simulink model "backup_of_step3"  (Simulink 10.2)
settings: Solver=ode113  StartTime=0.0  StopTime=5  RelTol=RT  AbsTol=AT  EnableMultiTasking=on
values from neighbouring files (symbols this model uses):
  Coefddq1 = polyfit(tv,ddq1d,5)    [TrajectoryPlanning_simulink.m]    (also in step2.mat = [4.72491967588e-15 -3.27046494167e-13 33.9277839628 -50.8916; step2_trajectory.m = polyfit(t_action,ddq1d,5); step3.m)
  Coefddq2 = polyfit(tv,ddq2d,5)    [TrajectoryPlanning_simulink.m]    (also in step2.mat = [9.35976668804e-13 -4.53899397056e-12 272.296235919 -408.444; step2_trajectory.m = polyfit(t_action,ddq2d,5); step3.m)
  Coefddq3 = polyfit(tv,ddq3d,5)    [TrajectoryPlanning_simulink.m]    (also in step2.mat = [-8.62483792285e-13 3.31083832504e-12 -180.560313738 270.840; step2_trajectory.m = polyfit(t_action,ddq3d,5); step3.m)
  Coefdq1 = polyfit(tv,dq1d,5)    [TrajectoryPlanning_simulink.m]    (also in step2.mat = [-5.68315943596e-14 8.48194599071 -16.9638919814 8.481945990; step2_trajectory.m = polyfit(t_action,dq1d,5); step3.m)
  Coefdq2 = polyfit(tv,dq2d,5)    [TrajectoryPlanning_simulink.m]    (also in step2.mat = [-5.14425222069e-13 68.0740589798 -136.14811796 68.074058979; step2_trajectory.m = polyfit(t_action,dq2d,5); step3.m)
  Coefdq3 = polyfit(tv,dq3d,5)    [TrajectoryPlanning_simulink.m]    (also in step2.mat = [8.05653713588e-13 -45.1400784346 90.2801568692 -45.14007843; step2_trajectory.m = polyfit(t_action,dq3d,5); step3.m)
  Coefq1 = polyfit(tv,q1d,5)    [TrajectoryPlanning_simulink.m]    (also in step2.mat = [1.69638919814 -4.24097299536 2.82731533024 7.50224544818e-1; step2_trajectory.m = polyfit(t_action,q1d,5); step3.m)
  Coefq2 = polyfit(tv,q2d,5)    [TrajectoryPlanning_simulink.m]    (also in step2.mat = [13.614811796 -34.0370294899 22.6913529933 -2.13681015439e-1; step2_trajectory.m = polyfit(t_action,q2d,5); step3.m)
  Coefq3 = polyfit(tv,q3d,5)    [TrajectoryPlanning_simulink.m]    (also in step2.mat = [-9.02801568692 22.5700392173 -15.0466928115 8.32884443522e-; step2_trajectory.m = polyfit(t_action,q3d,5); step3.m)
  F = [Fx;Fy;Mz]    [Jacobi_T.m]    (also in PRBDM_CTC_task.m = M_tilda*v+C_tilda*dX+G_tilda; RRR_CTC_task.m = M_tilda*v+V_tilda*dX+G_tilda; RRR_jtraj.m = q0; step2.mat = 10)
  gama0 = Rparams4dyn(3)    [PRBDM_3R_Dynamic_Matrices_Lagrange.m]    (also in PRBDM_3R_Dynamics.m = in4dyn(12); PRBDM_3R_Dynamics00.m = in4dyn(12); PRBDM_3R_DynamicsPID.m = in4dyn(12); PRBDM_3R_parameters.m = 0.1)
  gama1 = x(7)    [Jacobi_T.m]    (also in PRBDM_3R_Dynamic_Matrices_Lagrange.m = Rparams4dyn(4); PRBDM_3R_Dynamics.m = in4dyn(13); PRBDM_3R_Dynamics00.m = in4dyn(13); PRBDM_3R_DynamicsPID.m = in4dyn(13))
  gama2 = x(8)    [Jacobi_T.m]    (also in PRBDM_3R_Dynamic_Matrices_Lagrange.m = Rparams4dyn(5); PRBDM_3R_Dynamics.m = in4dyn(14); PRBDM_3R_Dynamics00.m = in4dyn(14); PRBDM_3R_DynamicsPID.m = in4dyn(14))
  gama3 = x(9)    [Jacobi_T.m]    (also in PRBDM_3R_Dynamic_Matrices_Lagrange.m = Rparams4dyn(6); PRBDM_3R_Dynamics.m = in4dyn(15); PRBDM_3R_Dynamics00.m = in4dyn(15); PRBDM_3R_DynamicsPID.m = in4dyn(15))
  k1 = Rparams4dyn(7)    [PRBDM_3R_Dynamic_Matrices_Lagrange.m]    (also in PRBDM_3R_Dynamics.m = in4dyn(16); PRBDM_3R_Dynamics00.m = in4dyn(16); PRBDM_3R_DynamicsPID.m = in4dyn(16); PRBDM_3R_parameters.m = 0.290628)
  k2 = Rparams4dyn(8)    [PRBDM_3R_Dynamic_Matrices_Lagrange.m]    (also in PRBDM_3R_Dynamics.m = in4dyn(17); PRBDM_3R_Dynamics00.m = in4dyn(17); PRBDM_3R_DynamicsPID.m = in4dyn(17); PRBDM_3R_parameters.m = 0.247572)
  k3 = Rparams4dyn(9)    [PRBDM_3R_Dynamic_Matrices_Lagrange.m]    (also in PRBDM_3R_Dynamics.m = in4dyn(18); PRBDM_3R_Dynamics00.m = in4dyn(18); PRBDM_3R_DynamicsPID.m = in4dyn(18); PRBDM_3R_parameters.m = 0.213624)
  kp = x(24)    [PRBDM_3R_CTC.m]    (also in PRBDM_3R_main.m = 20; PRBDM_3R_test001.m = 2; PRBDM_CTC_task.m = z(30); RRR_CTC.m)
  kv = x(23)    [PRBDM_3R_CTC.m]    (also in PRBDM_3R_main.m = 40; PRBDM_3R_test001.m = 4; PRBDM_CTC_task.m = z(29); RRR_CTC.m)
  L = Rparams4dyn(2)    [PRBDM_3R_Dynamic_Matrices_Lagrange.m]    (also in PRBDM_3R_Dynamics.m = in4dyn(11); PRBDM_3R_Dynamics00.m = in4dyn(11); PRBDM_3R_DynamicsPID.m = in4dyn(11); PRBDM_3R_parameters.m = 0.3)
  L0 = z(7)    [Forward_kinematics.m]    (also in GeometricCalculation_simulink.m = Geoparams(4); PRBDM_3R_parameters.m = 0.03; PRBDM_3R_parameters.mat = 0.03; TrajectoryPlanning_simulink.m = X(8))
  L1 = z(8)    [Forward_kinematics.m]    (also in GeometricCalculation_simulink.m = Geoparams(5); Jacobi.m = x(4); PRBDM_3R_CTC.m = x(19); PRBDM_3R_Dynamic_Matrices_NewtonEular.m = robot_params(4))
  L2 = z(9)    [Forward_kinematics.m]    (also in GeometricCalculation_simulink.m = Geoparams(6); Jacobi.m = x(5); PRBDM_3R_CTC.m = x(20); PRBDM_3R_Dynamic_Matrices_NewtonEular.m = robot_params(5))
  L3 = z(10)    [Forward_kinematics.m]    (also in GeometricCalculation_simulink.m = Geoparams(7); Jacobi.m = x(6); PRBDM_3R_CTC.m = x(21); PRBDM_3R_Dynamic_Matrices_NewtonEular.m = robot_params(6))
  m = Rparams4dyn(1)    [PRBDM_3R_Dynamic_Matrices_Lagrange.m]    (also in PRBDM_3R_Dynamics.m = in4dyn(10); PRBDM_3R_Dynamics00.m = in4dyn(10); PRBDM_3R_DynamicsPID.m = in4dyn(10); PRBDM_3R_parameters.m = 1)
  m1 = x(16)    [PRBDM_3R_CTC.m]    (also in PRBDM_3R_Dynamic_Matrices_NewtonEular.m = robot_params(1); PRBDM_3R_parameters.m = 0.35; PRBDM_3R_parameters.mat = 0.35; PRBDM_3R_test001.m = 0.1)
  m2 = x(17)    [PRBDM_3R_CTC.m]    (also in PRBDM_3R_Dynamic_Matrices_NewtonEular.m = robot_params(2); PRBDM_3R_parameters.m = 0.4; PRBDM_3R_parameters.mat = 0.4; PRBDM_3R_test001.m = 0.1)
  m3 = x(18)    [PRBDM_3R_CTC.m]    (also in PRBDM_3R_Dynamic_Matrices_NewtonEular.m = robot_params(3); PRBDM_3R_parameters.m = 0.15; PRBDM_3R_parameters.mat = 0.15; PRBDM_3R_test001.m = 0.1)
  Mz = x(6)    [Jacobi_T.m]    (also in step2.mat = 10; step2_trajectory.m = 10; step3.m = 10)
  phi = pi/3    (= 1.0471975512)    [PRBDM_3R_test001.m]
  t_action = [0 0.010101010101 0.020202020202 0.030303030303 0.040404040404 0.0505050505051 0.0606060606061 0.0707070707071 0.0808080808081 0.0909090909091 0.10101010101 0.111111111111 ... (100 elements, 1x100)]    [step2.mat]    (also in step2_trajectory.m = linspace(0,T_action,step); step3.m = 5)
  Theta_init = [0 0 0 0]    [step2.mat]    (also in step2_trajectory.m = [0     0     0     0    ]; step3.m = [0     0     0     0    ])
  W = x(22)    [PRBDM_3R_CTC.m]    (also in PRBDM_3R_Dynamic_Matrices_NewtonEular.m = robot_params(7); PRBDM_3R_Dynamics.m = in4dyn(20); PRBDM_3R_Dynamics00.m = in4dyn(20); PRBDM_3R_DynamicsPID.m = in4dyn(20))
  xd = 0.0536    [PRBDM_3R_test001.m]    (also in PRBDM_CTC_task.m = z(13); RRR_CTC_task.m = z(13))
  yd = 0.0135    [PRBDM_3R_test001.m]    (also in PRBDM_CTC_task.m = z(14); RRR_CTC_task.m = z(14))
settings Model: Creator=sayar  LastModifiedBy=Master
settings SolverCC: AutoScaleAbsTol=off
settings DataIOCC: SignalLoggingSaveFormat=Dataset  Refine=RF
settings OptimizationCC: ExpressionDepthLimit=2147483647
settings DebuggingCC: SolverPrmCheckMsg=warning  StateNameClashWarn=warning

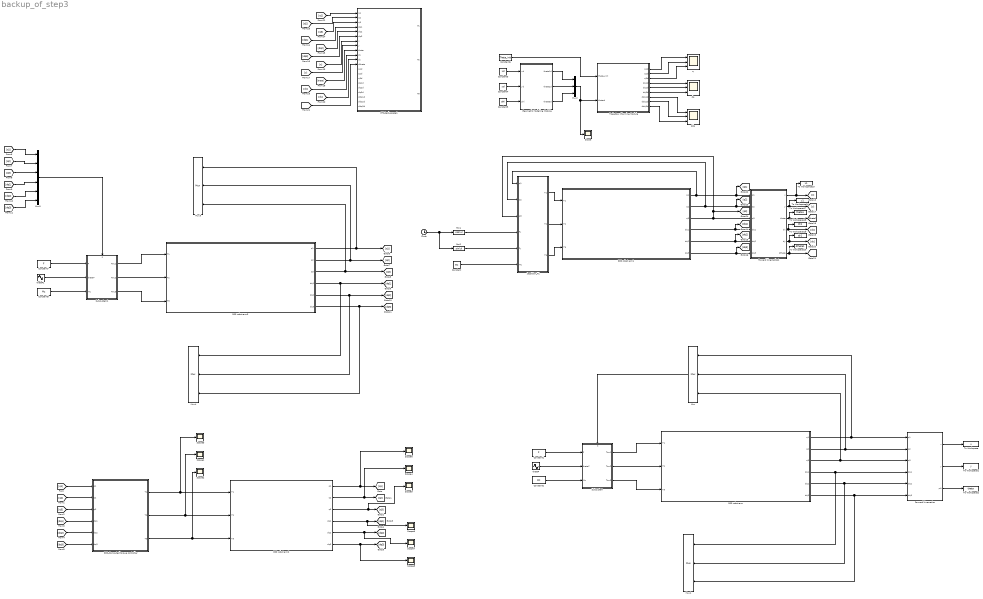
== system backup_of_step3 ==
  CTC_task_space1 : Subsystem
  Clock : Clock
  Constant : Constant  Value=Mz
  Constant1 : Constant  Value=F
  Constant2 : Constant  Value=Mz
  Constant3 : Constant  Value=xd
  Constant4 : Constant  Value=yd
  Constant5 : Constant  Value=phi
  Constant6 : Constant  Value=Theta_init
  Constant7 : Constant  Value=F
  Constant8 : Constant  Value=Mz
  Fcn1 : Fcn  Expr=cos(u)
  Fcn2 : Fcn  Expr=sin(u)
  Forward kinematics : Subsystem
  Forward kinematics1 : Subsystem
  Geometric Modeling Module : Subsystem
  Jacobian_T1 : Subsystem
  Mux{,1..4} (5 alike) : Mux  Inputs=3
  Mux5 : Mux  Inputs=6
  RRR robot arm : Subsystem
      mask Display: image(imread('RRR.png'))
  RRR robot arm1 : Subsystem
      mask Display: image(imread('RRR.png'))
  RRR robot arm2 : Subsystem
      mask Display: image(imread('RRR.png'))
  RRR robot arm3 : Subsystem
      mask Display: image(imread('RRR.png'))
  RRR_Computed torque controller : Subsystem
  Scope{,1..9} (10 alike) : Scope
  Subsystem : Subsystem
      settings: PortSchema="{\"entries\":[{\"content\":{\"sides\":[{\"content\":{\"connectorIds\":[\"In1\",\"In2\",\"In3\"]},\"type\":\"ConnectorPlacement.EquallySpacedRectSide\",\"uuid\":\"03e3fa68-98df-40a7-88fb-f274e89646de\"},{\"content\":{\"connectorIds\":[\"Out1\",\"Out2\",\"Out3\"],\"side\":\"RIGHT\"},\"type\":\"ConnectorPlacement.EquallySpacedRectSide\",\"uuid\":\"1a7c6e69-d785-4f03-b0d8-74a38f8f42a1\"},{\"content\":{\"connectorIds\":[\"In4\"],\"side\":\"TOP\"},\"type\":\"ConnectorPlacement.EquallySpacedRectSide\",\"uuid\":\"61c135cb-8cc5-493d-9c37-8230cda997e1\"},{\"content\":{\"connectorIds\":[],\"side\":\"HIDDEN\"},\"type\":\"ConnectorPlacement.EquallySpacedRectSide\",\"uuid\":\"5d99950e-feb6-474c-993a-cad470b06503\"}]},\"type\":\"ConnectorPlacement.EquallySpacedConnector\",\"uuid\":\"5533c5e9-db4a-4e3a-8115-8d67f8979e0c\"}],\"packageUris\":[\"http://schema.mathworks.com/mf0/Connector/R2020b\"],\"version\":\"1.0\"}"
  Subsystem1 : Subsystem
      settings: PortSchema="{\"entries\":[{\"content\":{\"sides\":[{\"content\":{\"connectorIds\":[\"In1\",\"In2\",\"In3\"]},\"type\":\"ConnectorPlacement.EquallySpacedRectSide\",\"uuid\":\"03e3fa68-98df-40a7-88fb-f274e89646de\"},{\"content\":{\"connectorIds\":[\"Out1\",\"Out2\",\"Out3\"],\"side\":\"RIGHT\"},\"type\":\"ConnectorPlacement.EquallySpacedRectSide\",\"uuid\":\"1a7c6e69-d785-4f03-b0d8-74a38f8f42a1\"},{\"content\":{\"connectorIds\":[\"In4\"],\"side\":\"TOP\"},\"type\":\"ConnectorPlacement.EquallySpacedRectSide\",\"uuid\":\"61c135cb-8cc5-493d-9c37-8230cda997e1\"},{\"content\":{\"connectorIds\":[],\"side\":\"HIDDEN\"},\"type\":\"ConnectorPlacement.EquallySpacedRectSide\",\"uuid\":\"5d99950e-feb6-474c-993a-cad470b06503\"}]},\"type\":\"ConnectorPlacement.EquallySpacedConnector\",\"uuid\":\"5533c5e9-db4a-4e3a-8115-8d67f8979e0c\"}],\"packageUris\":[\"http://schema.mathworks.com/mf0/Connector/R2020b\"],\"version\":\"1.0\"}"
  To Workspace : ToWorkspace  VariableName=x  SampleTime=-1
  To Workspace1 : ToWorkspace  VariableName=y  SampleTime=-1
  To Workspace15 : ToWorkspace  VariableName=x1  SampleTime=-1
  To Workspace16 : ToWorkspace  VariableName=y1  SampleTime=-1
  To Workspace17 : ToWorkspace  VariableName=theta1  SampleTime=-1
  To Workspace18 : ToWorkspace  VariableName=dx1  SampleTime=-1
  To Workspace19 : ToWorkspace  VariableName=dy1  SampleTime=-1
  To Workspace2 : ToWorkspace  VariableName=theta  SampleTime=-1
  To Workspace20 : ToWorkspace  VariableName=dtheta1  SampleTime=-1
  Trajectory Planning Module : Subsystem
  ddq : Scope  NumInputPorts=3
  dq : Scope  NumInputPorts=3
  q : Scope  NumInputPorts=3
  thetaF : Sin  SampleTime=0
  thetaF1 : Sin  SampleTime=0
  wires:
  Mux2/1 -> Scope/1, Trajectory Planning Module/2(thetad)
  Geometric Modeling Module/1(theta1d) -> Mux2/1
  Geometric Modeling Module/2(theta2d) -> Mux2/2
  Constant3/1 -> Geometric Modeling Module/1(xd)
  Constant5/1 -> Geometric Modeling Module/3(phi)
  Geometric Modeling Module/3(theta3d) -> Mux2/3
  Constant4/1 -> Geometric Modeling Module/2(yd)
  [y] -> CTC_task_space1/8(y)
  Forward kinematics1/6(dtheta) -> To Workspace20/1, [dtheta]
  Forward kinematics1/1(x) -> To Workspace15/1, [x]
  [dx] -> CTC_task_space1/10(dx)
  Forward kinematics1/3(theta) -> To Workspace17/1, [theta]
  RRR robot arm1/1(q1) -> [q1], Forward kinematics1/1(q1), Jacobian_T1/1(q1)
  [dy] -> CTC_task_space1/11(dy)
  RRR robot arm1/5(dq2) -> [dq2], Forward kinematics1/5(dq2)
  Jacobian_T1/3(T3) -> RRR robot arm1/3(T3)
  [dq2] -> CTC_task_space1/5(dq2)
  RRR robot arm1/6(dq3) -> [dq3], Forward kinematics1/6(dq3)
  [q1] -> CTC_task_space1/1(q1)
  [q3] -> CTC_task_space1/3(q3)
  [x] -> CTC_task_space1/7(x)
  [dq1] -> CTC_task_space1/4(dq1)
  Forward kinematics1/4(dx) -> To Workspace18/1, [dx]
  Forward kinematics1/2(y) -> To Workspace16/1, [y]
  Forward kinematics1/5(dy) -> To Workspace19/1, [dy]
  Jacobian_T1/2(T2) -> RRR robot arm1/2(T2)
  [dq3] -> CTC_task_space1/6(dq3)
  RRR robot arm1/4(dq1) -> [dq1], Forward kinematics1/4(dq1)
  [q2] -> CTC_task_space1/2(q2)
  Jacobian_T1/1(T1) -> RRR robot arm1/1(T1)
  RRR robot arm1/3(q3) -> Forward kinematics1/3(q3), [q3], Jacobian_T1/3(q3)
  [theta] -> CTC_task_space1/9(theta)
  [dtheta] -> CTC_task_space1/12(dtheta)
  RRR robot arm1/2(q2) -> [q2], Forward kinematics1/2(q2), Jacobian_T1/2(q2)
  Constant6/1 -> Trajectory Planning Module/1(theta_init)
  Trajectory Planning Module/1(q1d) -> q/1
  Trajectory Planning Module/2(q2d) -> q/2
  Trajectory Planning Module/3(q3d) -> q/3
  Trajectory Planning Module/4(dq1d) -> dq/1
  Trajectory Planning Module/5(dq2d) -> dq/2
  Trajectory Planning Module/6(dq3d) -> dq/3
  Trajectory Planning Module/8(ddq2d) -> ddq/2
  Trajectory Planning Module/9(ddq3d) -> ddq/3
  Trajectory Planning Module/7(ddq1d) -> ddq/1
  Clock/1 -> Fcn1/1, Fcn2/1
  Fcn2/1 -> Jacobian_T1/5(Fy)
  Fcn1/1 -> Jacobian_T1/4(Fx)
  Constant/1 -> Jacobian_T1/6(Mz)
  Mux/1 -> Subsystem/4(q)
  Subsystem/2(Tau2) -> RRR robot arm/2(T2)
  Subsystem/3(Tau3) -> RRR robot arm/3(T3)
  thetaF/1 -> Subsystem/2(thetaF)
  Forward kinematics/1(x) -> To Workspace/1
  Forward kinematics/3(phi) -> To Workspace2/1
  Forward kinematics/2(y) -> To Workspace1/1
  RRR robot arm/1(q1) -> Forward kinematics/1(q1), Mux/1
  Subsystem/1(Tau1) -> RRR robot arm/1(T1)
  RRR robot arm/2(q2) -> Mux/2, Forward kinematics/2(q2)
  RRR robot arm/6(dq3) -> Mux1/3, Forward kinematics/6(dq3)
  Constant2/1 -> Subsystem/3(Mz)
  RRR robot arm/5(dq2) -> Mux1/2, Forward kinematics/5(dq2)
  RRR robot arm/4(dq1) -> Mux1/1, Forward kinematics/4(dq1)
  RRR robot arm/3(q3) -> Mux/3, Forward kinematics/3(q3)
  Constant1/1 -> Subsystem/1(F)
  [dq3] -> RRR_Computed torque controller/6(dq3)
  RRR_Computed torque controller/1(T1) -> Scope3/1, RRR robot arm2/1(T1)
  [q3] -> RRR_Computed torque controller/3(q3)
  RRR robot arm2/5(dq2) -> Scope7/1, [dq2]
  RRR_Computed torque controller/2(T2) -> Scope1/1, RRR robot arm2/2(T2)
  RRR robot arm2/2(q2) -> Scope4/1, [q2]
  RRR robot arm2/4(dq1) -> Scope9/1, [dq1]
  RRR robot arm2/1(q1) -> Scope6/1, [q1]
  [dq1] -> RRR_Computed torque controller/4(dq1)
  [q2] -> RRR_Computed torque controller/2(q2)
  RRR robot arm2/6(dq3) -> Scope8/1, [dq3]
  [q1] -> RRR_Computed torque controller/1(q1)
  RRR_Computed torque controller/3(T3) -> Scope2/1, RRR robot arm2/3(T3)
  [dq2] -> RRR_Computed torque controller/5(dq2)
  RRR robot arm2/3(q3) -> Scope5/1, [q3]
  [dq3] -> Mux5/6
  [dq2] -> Mux5/5
  [q2] -> Mux5/2
  Subsystem1/3(Tau3) -> RRR robot arm3/3(T3)
  Subsystem1/2(Tau2) -> RRR robot arm3/2(T2)
  thetaF1/1 -> Subsystem1/2(thetaF)
  RRR robot arm3/6(dq3) -> [dq3], Mux4/3
  RRR robot arm3/2(q2) -> [q2], Mux3/2
  RRR robot arm3/1(q1) -> [q1], Mux3/1
  Subsystem1/1(Tau1) -> RRR robot arm3/1(T1)
  Constant7/1 -> Subsystem1/1(F)
  Constant8/1 -> Subsystem1/3(Mz)
  [q3] -> Mux5/3
  RRR robot arm3/5(dq2) -> [dq2], Mux4/2
  RRR robot arm3/4(dq1) -> [dq1], Mux4/1
  [q1] -> Mux5/1
  Mux5/1 -> Subsystem1/4(q)
  RRR robot arm3/3(q3) -> [q3], Mux3/3
  [dq1] -> Mux5/4

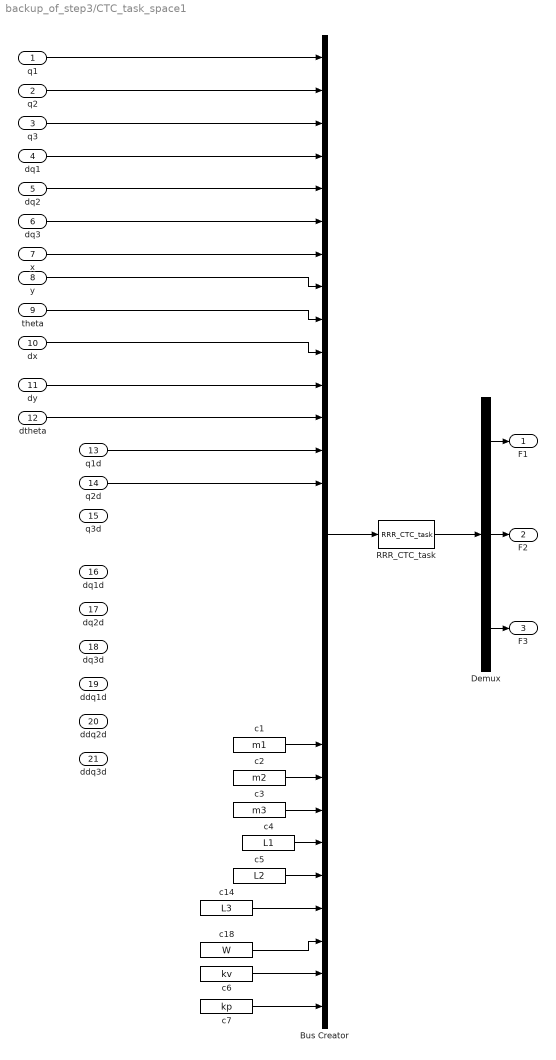
== system backup_of_step3/CTC_task_space1 ==
  q1 : Inport
  q2 : Inport  Port=2
  q3 : Inport  Port=3
  dq1 : Inport  Port=4
  dq2 : Inport  Port=5
  dq3 : Inport  Port=6
  x : Inport  Port=7
  y : Inport  Port=8
  theta : Inport  Port=9
  dx : Inport  Port=10
  dy : Inport  Port=11
  dtheta : Inport  Port=12
  q1d : Inport  Port=13
  q2d : Inport  Port=14
  q3d : Inport  Port=15
  dq1d : Inport  Port=16
  dq2d : Inport  Port=17
  dq3d : Inport  Port=18
  ddq1d : Inport  Port=19
  ddq2d : Inport  Port=20
  ddq3d : Inport  Port=21
  Bus Creator : BusCreator  Inputs=30
  Demux : Demux  Outputs=3
  RRR_CTC_task : MATLABFcn  MATLABFcn=RRR_CTC_task  OutputDimensions=3
  c1 : Constant  Value=m1
  c14 : Constant  Value=L3
  c18 : Constant  Value=W
  c2 : Constant  Value=m2
  c3 : Constant  Value=m3
  c4 : Constant  Value=L1
  c5 : Constant  Value=L2
  c6 : Constant  Value=kv
  c7 : Constant  Value=kp
  F1 : Outport
  F2 : Outport  Port=2
  F3 : Outport  Port=3
  wires:
  q3/1 -> Bus Creator/3
  RRR_CTC_task/1 -> Demux/1
  q1/1 -> Bus Creator/1
  Demux/3 -> F3/1
  q2/1 -> Bus Creator/2
  dq2/1 -> Bus Creator/5
  dq1/1 -> Bus Creator/4
  Demux/2 -> F2/1
  dq3/1 -> Bus Creator/6
  Demux/1 -> F1/1
  Bus Creator/1 -> RRR_CTC_task/1
  x/1 -> Bus Creator/7
  y/1 -> Bus Creator/8
  theta/1 -> Bus Creator/9
  dx/1 -> Bus Creator/10
  dy/1 -> Bus Creator/11
  dtheta/1 -> Bus Creator/12
  c1/1 -> Bus Creator/22
  c2/1 -> Bus Creator/23
  c3/1 -> Bus Creator/24
  c4/1 -> Bus Creator/25
  c5/1 -> Bus Creator/26
  c14/1 -> Bus Creator/27
  c18/1 -> Bus Creator/28
  c6/1 -> Bus Creator/29
  c7/1 -> Bus Creator/30
  q1d/1 -> Bus Creator/13
  q2d/1 -> Bus Creator/14

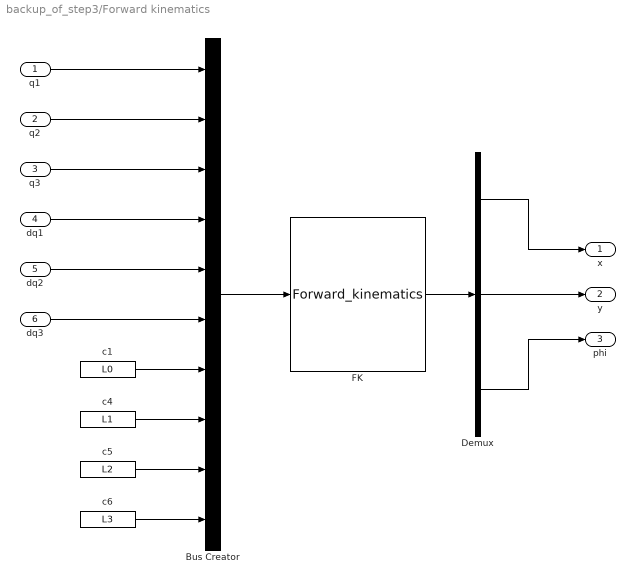
== system backup_of_step3/Forward kinematics ==
  q1 : Inport
  q2 : Inport  Port=2
  q3 : Inport  Port=3
  dq1 : Inport  Port=4
  dq2 : Inport  Port=5
  dq3 : Inport  Port=6
  Bus Creator : BusCreator  Inputs=10
  Demux : Demux  Outputs=3
  FK : MATLABFcn  MATLABFcn=Forward_kinematics  OutputDimensions=3
  c1 : Constant  Value=L0
  c4 : Constant  Value=L1
  c5 : Constant  Value=L2
  c6 : Constant  Value=L3
  x : Outport
  y : Outport  Port=2
  phi : Outport  Port=3
  wires:
  c6/1 -> Bus Creator/10
  Demux/1 -> x/1
  c4/1 -> Bus Creator/8
  q2/1 -> Bus Creator/2
  q1/1 -> Bus Creator/1
  q3/1 -> Bus Creator/3
  Bus Creator/1 -> FK/1
  dq2/1 -> Bus Creator/5
  Demux/2 -> y/1
  FK/1 -> Demux/1
  dq1/1 -> Bus Creator/4
  Demux/3 -> phi/1
  dq3/1 -> Bus Creator/6
  c5/1 -> Bus Creator/9
  c1/1 -> Bus Creator/7

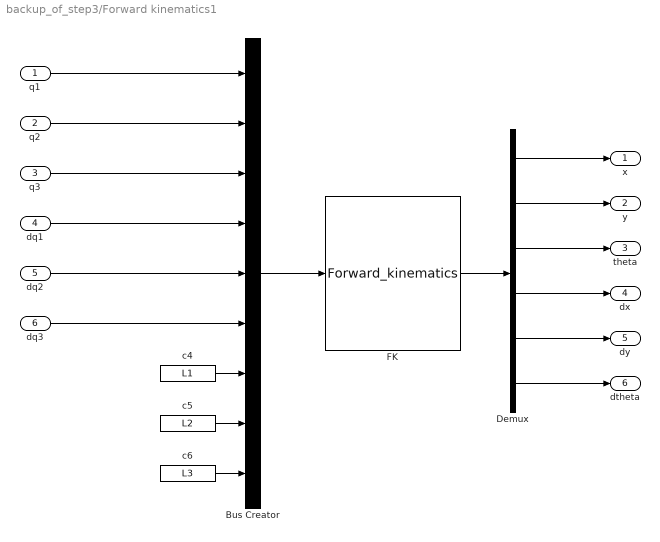
== system backup_of_step3/Forward kinematics1 ==
  q1 : Inport
  q2 : Inport  Port=2
  q3 : Inport  Port=3
  dq1 : Inport  Port=4
  dq2 : Inport  Port=5
  dq3 : Inport  Port=6
  Bus Creator : BusCreator  Inputs=9
  Demux : Demux  Outputs=6
  FK : MATLABFcn  MATLABFcn=Forward_kinematics  OutputDimensions=6
  c4 : Constant  Value=L1
  c5 : Constant  Value=L2
  c6 : Constant  Value=L3
  x : Outport
  y : Outport  Port=2
  theta : Outport  Port=3
  dx : Outport  Port=4
  dy : Outport  Port=5
  dtheta : Outport  Port=6
  wires:
  c6/1 -> Bus Creator/9
  Demux/1 -> x/1
  Demux/4 -> dx/1
  c4/1 -> Bus Creator/7
  Demux/5 -> dy/1
  q2/1 -> Bus Creator/2
  q1/1 -> Bus Creator/1
  q3/1 -> Bus Creator/3
  Bus Creator/1 -> FK/1
  dq2/1 -> Bus Creator/5
  Demux/2 -> y/1
  FK/1 -> Demux/1
  dq1/1 -> Bus Creator/4
  Demux/3 -> theta/1
  dq3/1 -> Bus Creator/6
  Demux/6 -> dtheta/1
  c5/1 -> Bus Creator/8

== system backup_of_step3/Geometric Modeling Module ==
  xd : Inport
  yd : Inport  Port=2
  phi : Inport  Port=3
  Demux : Demux  Outputs=3
  GeometricCalculation : MATLABFcn  MATLABFcn=GeometricCalculation_simulink
  Mux1 : Mux  Inputs=6
  c1 : Constant  Value=L0
  c2 : Constant  Value=L1
  c3 : Constant  Value=L2
  theta1d : Outport
  theta2d : Outport  Port=2
  theta3d : Outport  Port=3
  wires:
  Mux1/1 -> GeometricCalculation/1
  yd/1 -> Mux1/2
  xd/1 -> Mux1/1
  phi/1 -> Mux1/3
  c1/1 -> Mux1/4
  c3/1 -> Mux1/6
  c2/1 -> Mux1/5
  GeometricCalculation/1 -> Demux/1
  Demux/2 -> theta2d/1
  Demux/1 -> theta1d/1
  Demux/3 -> theta3d/1

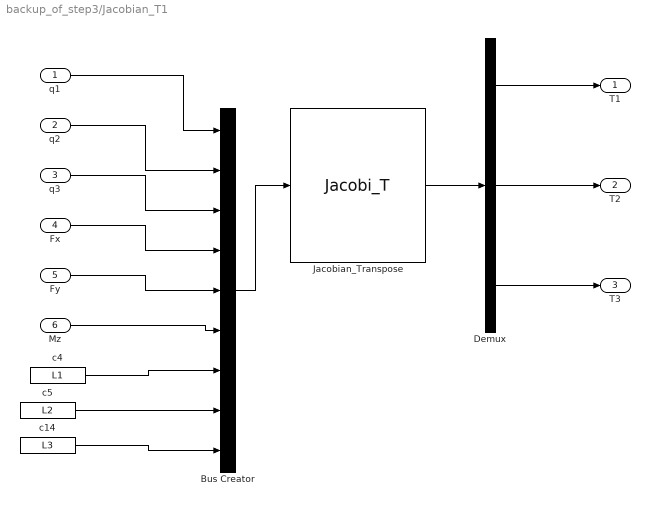
== system backup_of_step3/Jacobian_T1 ==
  q1 : Inport
  q2 : Inport  Port=2
  q3 : Inport  Port=3
  Fx : Inport  Port=4
  Fy : Inport  Port=5
  Mz : Inport  Port=6
  Bus Creator : BusCreator  Inputs=9
  Demux : Demux  Outputs=3
  Jacobian_Transpose : MATLABFcn  MATLABFcn=Jacobi_T  OutputDimensions=3
  c14 : Constant  Value=L3
  c4 : Constant  Value=L1
  c5 : Constant  Value=L2
  T1 : Outport
  T2 : Outport  Port=2
  T3 : Outport  Port=3
  wires:
  Jacobian_Transpose/1 -> Demux/1
  Demux/2 -> T2/1
  Bus Creator/1 -> Jacobian_Transpose/1
  Demux/1 -> T1/1
  Demux/3 -> T3/1
  Fx/1 -> Bus Creator/4
  Fy/1 -> Bus Creator/5
  Mz/1 -> Bus Creator/6
  q1/1 -> Bus Creator/1
  q2/1 -> Bus Creator/2
  q3/1 -> Bus Creator/3
  c5/1 -> Bus Creator/8
  c14/1 -> Bus Creator/9
  c4/1 -> Bus Creator/7

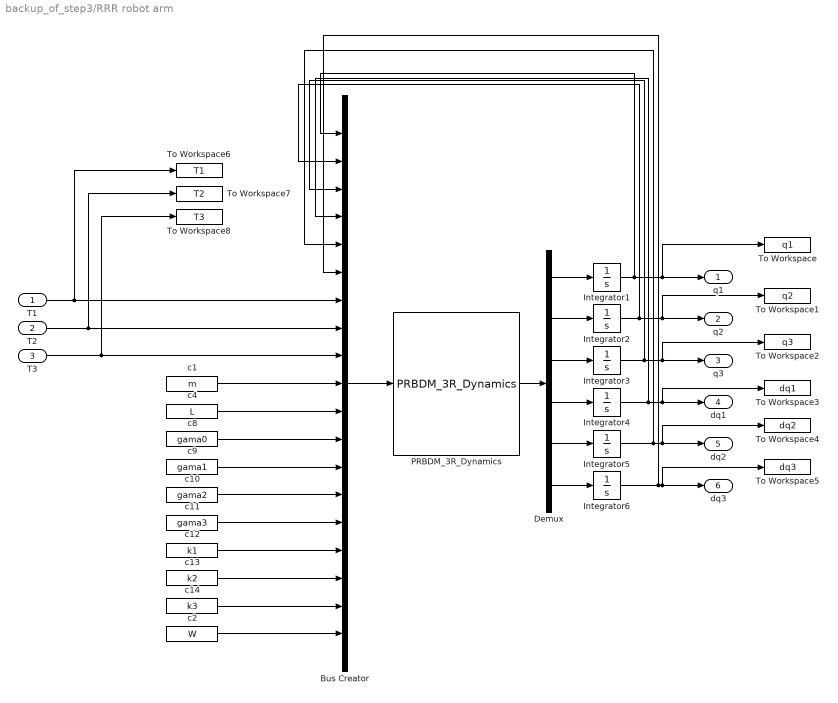
== system backup_of_step3/RRR robot arm ==
  T1 : Inport
  T2 : Inport  Port=2
  T3 : Inport  Port=3
  Bus Creator : BusCreator  Inputs=19
  Demux : Demux  Outputs=6
  Integrator{1,4..6} (4 alike) : Integrator
  Integrator2 : Integrator  InitialCondition=3*pi/4
  Integrator3 : Integrator  InitialCondition=-3*pi/4
  PRBDM_3R_Dynamics : MATLABFcn  MATLABFcn=PRBDM_3R_Dynamics  OutputDimensions=6
  To Workspace : ToWorkspace  VariableName=q1  SampleTime=-1
  To Workspace1 : ToWorkspace  VariableName=q2  SampleTime=-1
  To Workspace2 : ToWorkspace  VariableName=q3  SampleTime=-1
  To Workspace3 : ToWorkspace  VariableName=dq1  SampleTime=-1
  To Workspace4 : ToWorkspace  VariableName=dq2  SampleTime=-1
  To Workspace5 : ToWorkspace  VariableName=dq3  SampleTime=-1
  To Workspace6 : ToWorkspace  VariableName=T1  SampleTime=-1
  To Workspace7 : ToWorkspace  VariableName=T2  SampleTime=-1
  To Workspace8 : ToWorkspace  VariableName=T3  SampleTime=-1
  c1 : Constant  Value=m
  c10 : Constant  Value=gama2
  c11 : Constant  Value=gama3
  c12 : Constant  Value=k1
  c13 : Constant  Value=k2
  c14 : Constant  Value=k3
  c2 : Constant  Value=W
  c4 : Constant  Value=L
  c8 : Constant  Value=gama0
  c9 : Constant  Value=gama1
  q1 : Outport
  q2 : Outport  Port=2
  q3 : Outport  Port=3
  dq1 : Outport  Port=4
  dq2 : Outport  Port=5
  dq3 : Outport  Port=6
  wires:
  Demux/1 -> Integrator1/1
  Demux/2 -> Integrator2/1
  Demux/3 -> Integrator3/1
  Demux/4 -> Integrator4/1
  Demux/5 -> Integrator5/1
  Demux/6 -> Integrator6/1
  Integrator1/1 -> Bus Creator/1, q1/1, To Workspace/1
  Integrator2/1 -> Bus Creator/2, q2/1, To Workspace1/1
  Integrator3/1 -> Bus Creator/3, q3/1, To Workspace2/1
  Integrator4/1 -> Bus Creator/4, dq1/1, To Workspace3/1
  Integrator5/1 -> Bus Creator/5, dq2/1, To Workspace4/1
  Integrator6/1 -> Bus Creator/6, dq3/1, To Workspace5/1
  c1/1 -> Bus Creator/10
  PRBDM_3R_Dynamics/1 -> Demux/1
  Bus Creator/1 -> PRBDM_3R_Dynamics/1
  T3/1 -> To Workspace8/1, Bus Creator/9
  T2/1 -> To Workspace7/1, Bus Creator/8
  T1/1 -> To Workspace6/1, Bus Creator/7
  c4/1 -> Bus Creator/11
  c8/1 -> Bus Creator/12
  c9/1 -> Bus Creator/13
  c10/1 -> Bus Creator/14
  c11/1 -> Bus Creator/15
  c12/1 -> Bus Creator/16
  c13/1 -> Bus Creator/17
  c14/1 -> Bus Creator/18
  c2/1 -> Bus Creator/19

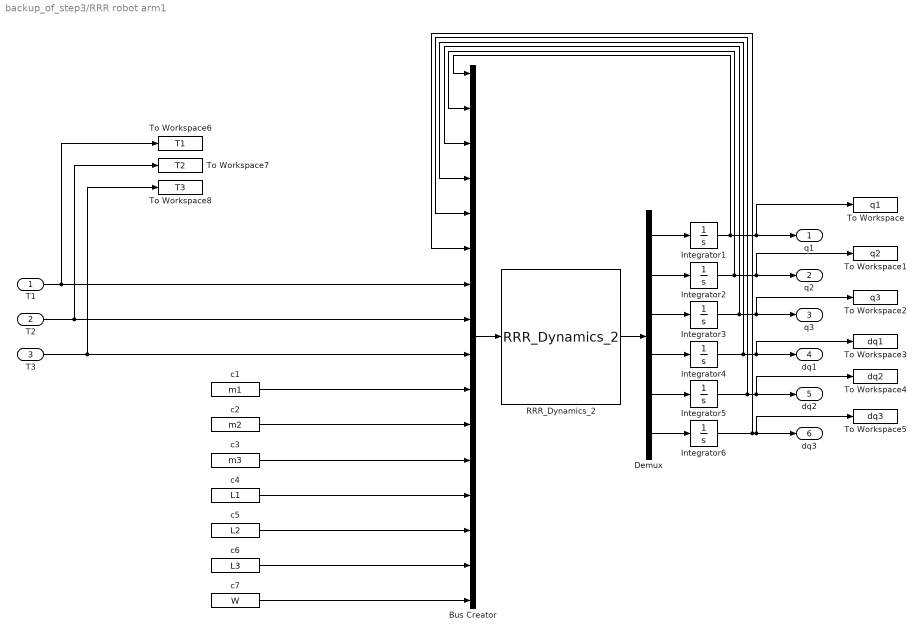
== system backup_of_step3/RRR robot arm1 ==
  T1 : Inport
  T2 : Inport  Port=2
  T3 : Inport  Port=3
  Bus Creator : BusCreator  Inputs=16
  Demux : Demux  Outputs=6
  Integrator{1,4..6} (4 alike) : Integrator
  Integrator2 : Integrator  InitialCondition=3*pi/4
  Integrator3 : Integrator  InitialCondition=-3*pi/4
  RRR_Dynamics_2 : MATLABFcn  MATLABFcn=RRR_Dynamics_2  OutputDimensions=6
  To Workspace : ToWorkspace  VariableName=q1  SampleTime=-1
  To Workspace1 : ToWorkspace  VariableName=q2  SampleTime=-1
  To Workspace2 : ToWorkspace  VariableName=q3  SampleTime=-1
  To Workspace3 : ToWorkspace  VariableName=dq1  SampleTime=-1
  To Workspace4 : ToWorkspace  VariableName=dq2  SampleTime=-1
  To Workspace5 : ToWorkspace  VariableName=dq3  SampleTime=-1
  To Workspace6 : ToWorkspace  VariableName=T1  SampleTime=-1
  To Workspace7 : ToWorkspace  VariableName=T2  SampleTime=-1
  To Workspace8 : ToWorkspace  VariableName=T3  SampleTime=-1
  c1 : Constant  Value=m1
  c2 : Constant  Value=m2
  c3 : Constant  Value=m3
  c4 : Constant  Value=L1
  c5 : Constant  Value=L2
  c6 : Constant  Value=L3
  c7 : Constant  Value=W
  q1 : Outport
  q2 : Outport  Port=2
  q3 : Outport  Port=3
  dq1 : Outport  Port=4
  dq2 : Outport  Port=5
  dq3 : Outport  Port=6
  wires:
  Demux/1 -> Integrator1/1
  Demux/2 -> Integrator2/1
  Demux/3 -> Integrator3/1
  Demux/4 -> Integrator4/1
  Demux/5 -> Integrator5/1
  Demux/6 -> Integrator6/1
  Integrator1/1 -> Bus Creator/1, q1/1, To Workspace/1
  Integrator2/1 -> Bus Creator/2, q2/1, To Workspace1/1
  Integrator3/1 -> Bus Creator/3, q3/1, To Workspace2/1
  Integrator4/1 -> Bus Creator/4, dq1/1, To Workspace3/1
  Integrator5/1 -> Bus Creator/5, dq2/1, To Workspace4/1
  Integrator6/1 -> Bus Creator/6, dq3/1, To Workspace5/1
  c1/1 -> Bus Creator/10
  c2/1 -> Bus Creator/11
  RRR_Dynamics_2/1 -> Demux/1
  Bus Creator/1 -> RRR_Dynamics_2/1
  T3/1 -> To Workspace8/1, Bus Creator/9
  T2/1 -> To Workspace7/1, Bus Creator/8
  T1/1 -> To Workspace6/1, Bus Creator/7
  c3/1 -> Bus Creator/12
  c4/1 -> Bus Creator/13
  c5/1 -> Bus Creator/14
  c6/1 -> Bus Creator/15
  c7/1 -> Bus Creator/16

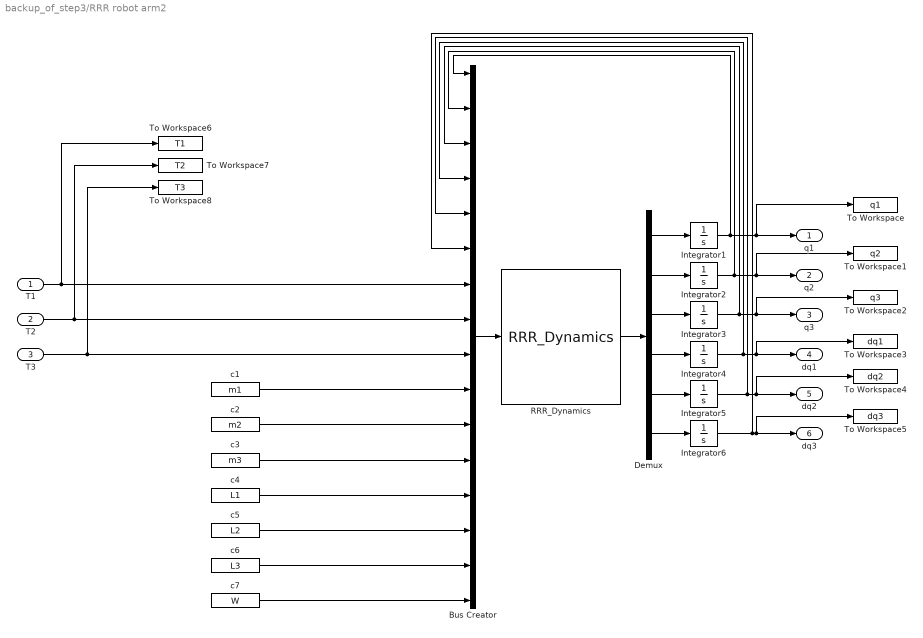
== system backup_of_step3/RRR robot arm2 ==
  T1 : Inport
  T2 : Inport  Port=2
  T3 : Inport  Port=3
  Bus Creator : BusCreator  Inputs=16
  Demux : Demux  Outputs=6
  Integrator{1,4..6} (4 alike) : Integrator
  Integrator2 : Integrator  InitialCondition=3*pi/4
  Integrator3 : Integrator  InitialCondition=-3*pi/4
  RRR_Dynamics : MATLABFcn  MATLABFcn=RRR_Dynamics  OutputDimensions=6
  To Workspace : ToWorkspace  VariableName=q1  SampleTime=-1
  To Workspace1 : ToWorkspace  VariableName=q2  SampleTime=-1
  To Workspace2 : ToWorkspace  VariableName=q3  SampleTime=-1
  To Workspace3 : ToWorkspace  VariableName=dq1  SampleTime=-1
  To Workspace4 : ToWorkspace  VariableName=dq2  SampleTime=-1
  To Workspace5 : ToWorkspace  VariableName=dq3  SampleTime=-1
  To Workspace6 : ToWorkspace  VariableName=T1  SampleTime=-1
  To Workspace7 : ToWorkspace  VariableName=T2  SampleTime=-1
  To Workspace8 : ToWorkspace  VariableName=T3  SampleTime=-1
  c1 : Constant  Value=m1
  c2 : Constant  Value=m2
  c3 : Constant  Value=m3
  c4 : Constant  Value=L1
  c5 : Constant  Value=L2
  c6 : Constant  Value=L3
  c7 : Constant  Value=W
  q1 : Outport
  q2 : Outport  Port=2
  q3 : Outport  Port=3
  dq1 : Outport  Port=4
  dq2 : Outport  Port=5
  dq3 : Outport  Port=6
  wires:
  Demux/1 -> Integrator1/1
  Demux/2 -> Integrator2/1
  Demux/3 -> Integrator3/1
  Demux/4 -> Integrator4/1
  Demux/5 -> Integrator5/1
  Demux/6 -> Integrator6/1
  Integrator1/1 -> Bus Creator/1, q1/1, To Workspace/1
  Integrator2/1 -> Bus Creator/2, q2/1, To Workspace1/1
  Integrator3/1 -> Bus Creator/3, q3/1, To Workspace2/1
  Integrator4/1 -> Bus Creator/4, dq1/1, To Workspace3/1
  Integrator5/1 -> Bus Creator/5, dq2/1, To Workspace4/1
  Integrator6/1 -> Bus Creator/6, dq3/1, To Workspace5/1
  c1/1 -> Bus Creator/10
  c2/1 -> Bus Creator/11
  RRR_Dynamics/1 -> Demux/1
  Bus Creator/1 -> RRR_Dynamics/1
  T3/1 -> To Workspace8/1, Bus Creator/9
  T2/1 -> To Workspace7/1, Bus Creator/8
  T1/1 -> To Workspace6/1, Bus Creator/7
  c3/1 -> Bus Creator/12
  c4/1 -> Bus Creator/13
  c5/1 -> Bus Creator/14
  c6/1 -> Bus Creator/15
  c7/1 -> Bus Creator/16

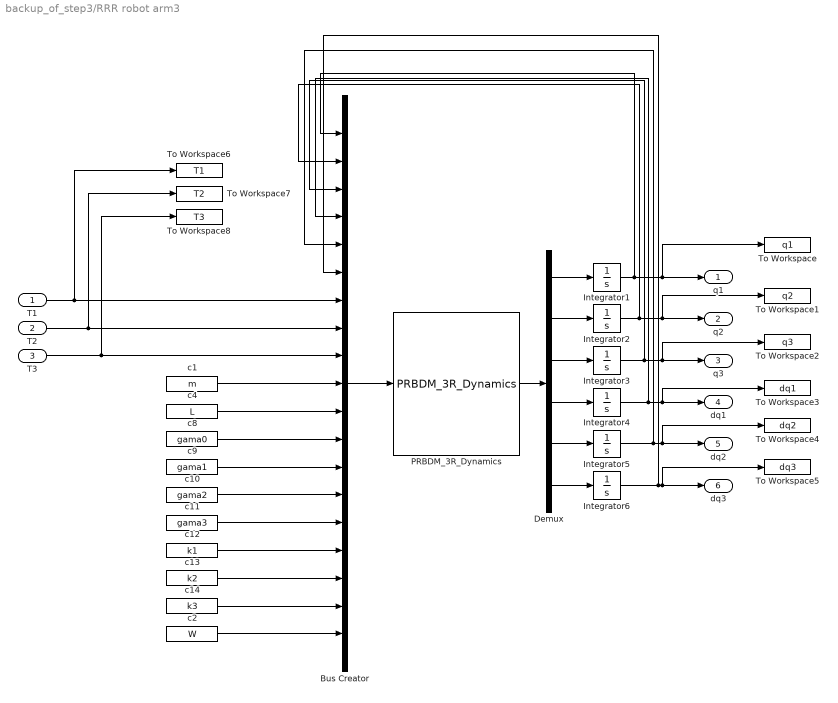
== system backup_of_step3/RRR robot arm3 ==
  T1 : Inport
  T2 : Inport  Port=2
  T3 : Inport  Port=3
  Bus Creator : BusCreator  Inputs=19
  Demux : Demux  Outputs=6
  Integrator{1,4..6} (4 alike) : Integrator
  Integrator2 : Integrator  InitialCondition=3*pi/4
  Integrator3 : Integrator  InitialCondition=-3*pi/4
  PRBDM_3R_Dynamics : MATLABFcn  MATLABFcn=PRBDM_3R_Dynamics  OutputDimensions=6
  To Workspace : ToWorkspace  VariableName=q1  SampleTime=-1
  To Workspace1 : ToWorkspace  VariableName=q2  SampleTime=-1
  To Workspace2 : ToWorkspace  VariableName=q3  SampleTime=-1
  To Workspace3 : ToWorkspace  VariableName=dq1  SampleTime=-1
  To Workspace4 : ToWorkspace  VariableName=dq2  SampleTime=-1
  To Workspace5 : ToWorkspace  VariableName=dq3  SampleTime=-1
  To Workspace6 : ToWorkspace  VariableName=T1  SampleTime=-1
  To Workspace7 : ToWorkspace  VariableName=T2  SampleTime=-1
  To Workspace8 : ToWorkspace  VariableName=T3  SampleTime=-1
  c1 : Constant  Value=m
  c10 : Constant  Value=gama2
  c11 : Constant  Value=gama3
  c12 : Constant  Value=k1
  c13 : Constant  Value=k2
  c14 : Constant  Value=k3
  c2 : Constant  Value=W
  c4 : Constant  Value=L
  c8 : Constant  Value=gama0
  c9 : Constant  Value=gama1
  q1 : Outport
  q2 : Outport  Port=2
  q3 : Outport  Port=3
  dq1 : Outport  Port=4
  dq2 : Outport  Port=5
  dq3 : Outport  Port=6
  wires:
  Demux/1 -> Integrator1/1
  Demux/2 -> Integrator2/1
  Demux/3 -> Integrator3/1
  Demux/4 -> Integrator4/1
  Demux/5 -> Integrator5/1
  Demux/6 -> Integrator6/1
  Integrator1/1 -> Bus Creator/1, q1/1, To Workspace/1
  Integrator2/1 -> Bus Creator/2, q2/1, To Workspace1/1
  Integrator3/1 -> Bus Creator/3, q3/1, To Workspace2/1
  Integrator4/1 -> Bus Creator/4, dq1/1, To Workspace3/1
  Integrator5/1 -> Bus Creator/5, dq2/1, To Workspace4/1
  Integrator6/1 -> Bus Creator/6, dq3/1, To Workspace5/1
  c1/1 -> Bus Creator/10
  PRBDM_3R_Dynamics/1 -> Demux/1
  Bus Creator/1 -> PRBDM_3R_Dynamics/1
  T3/1 -> To Workspace8/1, Bus Creator/9
  T2/1 -> To Workspace7/1, Bus Creator/8
  T1/1 -> To Workspace6/1, Bus Creator/7
  c4/1 -> Bus Creator/11
  c8/1 -> Bus Creator/12
  c9/1 -> Bus Creator/13
  c10/1 -> Bus Creator/14
  c11/1 -> Bus Creator/15
  c12/1 -> Bus Creator/16
  c13/1 -> Bus Creator/17
  c14/1 -> Bus Creator/18
  c2/1 -> Bus Creator/19

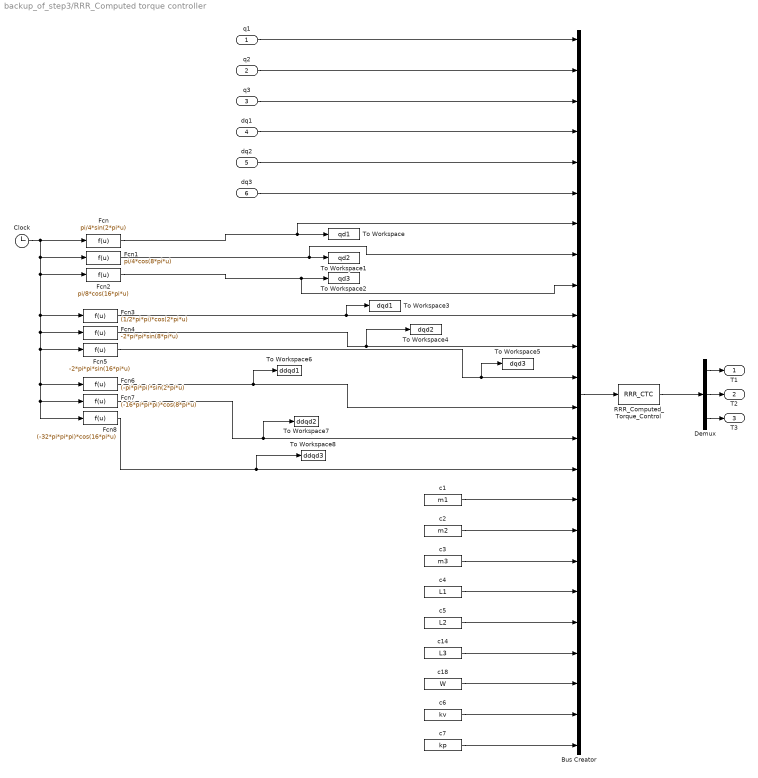
== system backup_of_step3/RRR_Computed torque controller ==
  q1 : Inport
  q2 : Inport  Port=2
  q3 : Inport  Port=3
  dq1 : Inport  Port=4
  dq2 : Inport  Port=5
  dq3 : Inport  Port=6
  Bus Creator : BusCreator  Inputs=24
  Clock : Clock
  Demux : Demux  Outputs=3
  Fcn : Fcn  Expr=pi/4*sin(2*pi*u)
  Fcn1 : Fcn  Expr=pi/4*cos(8*pi*u)
  Fcn2 : Fcn  Expr=pi/8*cos(16*pi*u)
  Fcn3 : Fcn  Expr=(1/2*pi*pi)*cos(2*pi*u)
  Fcn4 : Fcn  Expr=-2*pi*pi*sin(8*pi*u)
  Fcn5 : Fcn  Expr=-2*pi*pi*sin(16*pi*u)
  Fcn6 : Fcn  Expr=(-pi*pi*pi)*sin(2*pi*u)
  Fcn7 : Fcn  Expr=(-16*pi*pi*pi)*cos(8*pi*u)
  Fcn8 : Fcn  Expr=(-32*pi*pi*pi)*cos(16*pi*u)
  RRR_Computed_Torque_Control : MATLABFcn  MATLABFcn=RRR_CTC  OutputDimensions=3
  To Workspace : ToWorkspace  VariableName=qd1  SampleTime=-1
  To Workspace1 : ToWorkspace  VariableName=qd2  SampleTime=-1
  To Workspace2 : ToWorkspace  VariableName=qd3  SampleTime=-1
  To Workspace3 : ToWorkspace  VariableName=dqd1  SampleTime=-1
  To Workspace4 : ToWorkspace  VariableName=dqd2  SampleTime=-1
  To Workspace5 : ToWorkspace  VariableName=dqd3  SampleTime=-1
  To Workspace6 : ToWorkspace  VariableName=ddqd1  SampleTime=-1
  To Workspace7 : ToWorkspace  VariableName=ddqd2  SampleTime=-1
  To Workspace8 : ToWorkspace  VariableName=ddqd3  SampleTime=-1
  c1 : Constant  Value=m1
  c14 : Constant  Value=L3
  c18 : Constant  Value=W
  c2 : Constant  Value=m2
  c3 : Constant  Value=m3
  c4 : Constant  Value=L1
  c5 : Constant  Value=L2
  c6 : Constant  Value=kv
  c7 : Constant  Value=kp
  T1 : Outport
  T2 : Outport  Port=2
  T3 : Outport  Port=3
  wires:
  RRR_Computed_Torque_Control/1 -> Demux/1
  Bus Creator/1 -> RRR_Computed_Torque_Control/1
  Demux/1 -> T1/1
  Demux/2 -> T2/1
  Demux/3 -> T3/1
  c1/1 -> Bus Creator/16
  c2/1 -> Bus Creator/17
  c3/1 -> Bus Creator/18
  c14/1 -> Bus Creator/21
  c18/1 -> Bus Creator/22
  q1/1 -> Bus Creator/1
  q2/1 -> Bus Creator/2
  q3/1 -> Bus Creator/3
  dq1/1 -> Bus Creator/4
  dq2/1 -> Bus Creator/5
  dq3/1 -> Bus Creator/6
  Clock/1 -> Fcn5/1, Fcn8/1, Fcn7/1, Fcn6/1, Fcn4/1, Fcn3/1, Fcn2/1, Fcn1/1, Fcn/1
  Fcn/1 -> Bus Creator/7, To Workspace/1
  Fcn1/1 -> Bus Creator/8, To Workspace1/1
  Fcn2/1 -> Bus Creator/9, To Workspace2/1
  Fcn3/1 -> To Workspace3/1, Bus Creator/10
  Fcn4/1 -> To Workspace4/1, Bus Creator/11
  Fcn5/1 -> To Workspace5/1, Bus Creator/12
  Fcn6/1 -> To Workspace6/1, Bus Creator/13
  Fcn7/1 -> To Workspace7/1, Bus Creator/14
  Fcn8/1 -> To Workspace8/1, Bus Creator/15
  c4/1 -> Bus Creator/19
  c5/1 -> Bus Creator/20
  c6/1 -> Bus Creator/23
  c7/1 -> Bus Creator/24

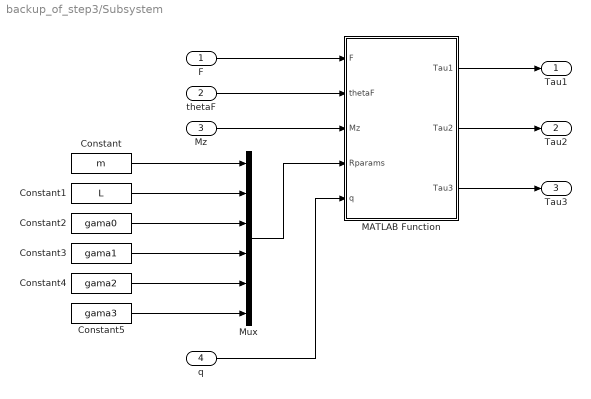
== system backup_of_step3/Subsystem ==
  F : Inport
  thetaF : Inport  Port=2
  Mz : Inport  Port=3
  q : Inport  Port=4
  Constant : Constant  Value=m
  Constant1 : Constant  Value=L
  Constant2 : Constant  Value=gama0
  Constant3 : Constant  Value=gama1
  Constant4 : Constant  Value=gama2
  Constant5 : Constant  Value=gama3
  MATLAB Function : MATLAB Function  TreatAsAtomicUnit=on
  Mux : Mux  Inputs=6
  Tau1 : Outport
  Tau2 : Outport  Port=2
  Tau3 : Outport  Port=3
  wires:
  thetaF/1 -> MATLAB Function/2(thetaF)
  F/1 -> MATLAB Function/1(F)
  Mz/1 -> MATLAB Function/3(Mz)
  MATLAB Function/1(Tau1) -> Tau1/1
  Constant/1 -> Mux/1
  Constant1/1 -> Mux/2
  Constant2/1 -> Mux/3
  Constant3/1 -> Mux/4
  Constant4/1 -> Mux/5
  Constant5/1 -> Mux/6
  Mux/1 -> MATLAB Function/4(Rparams)
  MATLAB Function/2(Tau2) -> Tau2/1
  MATLAB Function/3(Tau3) -> Tau3/1
  q/1 -> MATLAB Function/5(q)

== system backup_of_step3/Subsystem1 ==
  F : Inport
  thetaF : Inport  Port=2
  Mz : Inport  Port=3
  q : Inport  Port=4
  Constant : Constant  Value=m
  Constant1 : Constant  Value=L
  Constant2 : Constant  Value=gama0
  Constant3 : Constant  Value=gama1
  Constant4 : Constant  Value=gama2
  Constant5 : Constant  Value=gama3
  MATLAB Function : MATLAB Function  TreatAsAtomicUnit=on
  Mux : Mux  Inputs=6
  Tau1 : Outport
  Tau2 : Outport  Port=2
  Tau3 : Outport  Port=3
  wires:
  thetaF/1 -> MATLAB Function/2(thetaF)
  F/1 -> MATLAB Function/1(F)
  Mz/1 -> MATLAB Function/3(Mz)
  MATLAB Function/1(Tau1) -> Tau1/1
  Constant/1 -> Mux/1
  Constant1/1 -> Mux/2
  Constant2/1 -> Mux/3
  Constant3/1 -> Mux/4
  Constant4/1 -> Mux/5
  Constant5/1 -> Mux/6
  Mux/1 -> MATLAB Function/4(Rparams)
  MATLAB Function/2(Tau2) -> Tau2/1
  MATLAB Function/3(Tau3) -> Tau3/1
  q/1 -> MATLAB Function/5(q)

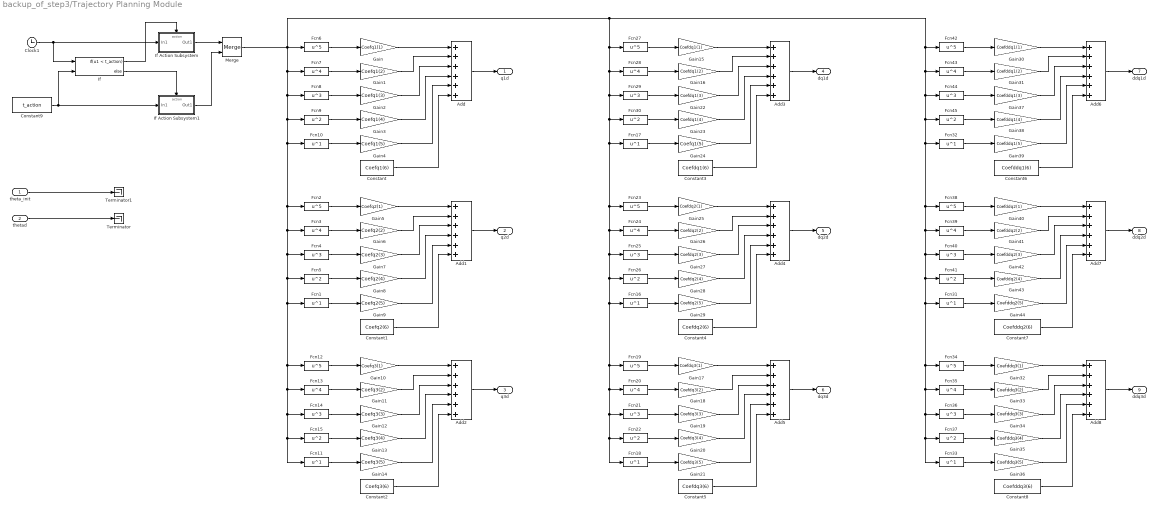
== system backup_of_step3/Trajectory Planning Module ==
  theta_init : Inport
  thetad : Inport  Port=2
  Add{,1..8} (9 alike) : Sum  Inputs=++++++
  Clock1 : Clock
  Constant : Constant  Value=Coefq1(6)
  Constant1 : Constant  Value=Coefq2(6)
  Constant2 : Constant  Value=Coefq3(6)
  Constant3 : Constant  Value=Coefdq1(6)
  Constant4 : Constant  Value=Coefdq2(6)
  Constant5 : Constant  Value=Coefdq3(6)
  Constant6 : Constant  Value=Coefddq1(6)
  Constant7 : Constant  Value=Coefddq2(6)
  Constant8 : Constant  Value=Coefddq3(6)
  Constant9 : Constant  Value=t_action
  Fcn{1,10..11,16..18,31..33} (9 alike) : Fcn  Expr=u^1
  Fcn{2,6,12,19,23,27,34,38,42} (9 alike) : Fcn  Expr=u^5
  Fcn{3,7,13,20,24,28,35,39,43} (9 alike) : Fcn  Expr=u^4
  Fcn{4,8,14,21,25,29,36,40,44} (9 alike) : Fcn  Expr=u^3
  Fcn{5,9,15,22,26,30,37,41,45} (9 alike) : Fcn  Expr=u^2
  Gain : Gain  Gain=Coefq1(1)
  Gain1 : Gain  Gain=Coefq1(2)
  Gain10 : Gain  Gain=Coefq3(1)
  Gain11 : Gain  Gain=Coefq3(2)
  Gain12 : Gain  Gain=Coefq3(3)
  Gain13 : Gain  Gain=Coefq3(4)
  Gain14 : Gain  Gain=Coefq3(5)
  Gain15 : Gain  Gain=Coefdq1(1)
  Gain16 : Gain  Gain=Coefdq1(2)
  Gain17 : Gain  Gain=Coefdq3(1)
  Gain18 : Gain  Gain=Coefdq3(2)
  Gain19 : Gain  Gain=Coefdq3(3)
  Gain2 : Gain  Gain=Coefq1(3)
  Gain20 : Gain  Gain=Coefdq3(4)
  Gain21 : Gain  Gain=Coefdq3(5)
  Gain22 : Gain  Gain=Coefdq1(3)
  Gain23 : Gain  Gain=Coefdq1(4)
  Gain24 : Gain  Gain=Coefq1(5)
  Gain25 : Gain  Gain=Coefdq2(1)
  Gain26 : Gain  Gain=Coefdq2(2)
  Gain27 : Gain  Gain=Coefdq2(3)
  Gain28 : Gain  Gain=Coefdq2(4)
  Gain29 : Gain  Gain=Coefdq2(5)
  Gain3 : Gain  Gain=Coefq1(4)
  Gain30 : Gain  Gain=Coefddq1(1)
  Gain31 : Gain  Gain=Coefddq1(2)
  Gain32 : Gain  Gain=Coefddq3(1)
  Gain33 : Gain  Gain=Coefddq3(2)
  Gain34 : Gain  Gain=Coefddq3(3)
  Gain35 : Gain  Gain=Coefddq3(4)
  Gain36 : Gain  Gain=Coefddq3(5)
  Gain37 : Gain  Gain=Coefddq1(3)
  Gain38 : Gain  Gain=Coefddq1(4)
  Gain39 : Gain  Gain=Coefddq1(5)
  Gain4 : Gain  Gain=Coefq1(5)
  Gain40 : Gain  Gain=Coefddq2(1)
  Gain41 : Gain  Gain=Coefddq2(2)
  Gain42 : Gain  Gain=Coefddq2(3)
  Gain43 : Gain  Gain=Coefddq2(4)
  Gain44 : Gain  Gain=Coefddq2(5)
  Gain5 : Gain  Gain=Coefq2(1)
  Gain6 : Gain  Gain=Coefq2(2)
  Gain7 : Gain  Gain=Coefq2(3)
  Gain8 : Gain  Gain=Coefq2(4)
  Gain9 : Gain  Gain=Coefq2(5)
  If : If  NumInputs=2  IfExpression=u1 < t_action
  If Action Subsystem : Subsystem  TreatAsAtomicUnit=on
  If Action Subsystem1 : Subsystem  TreatAsAtomicUnit=on
  Merge : Merge
  Terminator : Terminator
  Terminator1 : Terminator
  q1d : Outport
  q2d : Outport  Port=2
  q3d : Outport  Port=3
  dq1d : Outport  Port=4
  dq2d : Outport  Port=5
  dq3d : Outport  Port=6
  ddq1d : Outport  Port=7
  ddq2d : Outport  Port=8
  ddq3d : Outport  Port=9
  wires:
  Clock1/1 -> If/1, If Action Subsystem/1(In1)
  Fcn6/1 -> Gain/1
  Fcn8/1 -> Gain2/1
  Fcn7/1 -> Gain1/1
  Fcn9/1 -> Gain3/1
  Fcn10/1 -> Gain4/1
  Gain/1 -> Add/1
  Gain1/1 -> Add/2
  Gain2/1 -> Add/3
  Gain3/1 -> Add/4
  Gain4/1 -> Add/5
  Constant/1 -> Add/6
  Add/1 -> q1d/1
  Add1/1 -> q2d/1
  Fcn2/1 -> Gain5/1
  Fcn5/1 -> Gain8/1
  Gain6/1 -> Add1/2
  Gain9/1 -> Add1/5
  Constant1/1 -> Add1/6
  Fcn1/1 -> Gain9/1
  Gain8/1 -> Add1/4
  Gain5/1 -> Add1/1
  Fcn3/1 -> Gain6/1
  Fcn4/1 -> Gain7/1
  Gain7/1 -> Add1/3
  Gain11/1 -> Add2/2
  Fcn12/1 -> Gain10/1
  Fcn15/1 -> Gain13/1
  Gain14/1 -> Add2/5
  Fcn13/1 -> Gain11/1
  Gain10/1 -> Add2/1
  Fcn14/1 -> Gain12/1
  Constant2/1 -> Add2/6
  Gain13/1 -> Add2/4
  Fcn11/1 -> Gain14/1
  Gain12/1 -> Add2/3
  Add2/1 -> q3d/1
  Fcn21/1 -> Gain19/1
  Gain19/1 -> Add5/3
  Gain20/1 -> Add5/4
  Fcn18/1 -> Gain21/1
  Gain21/1 -> Add5/5
  Gain18/1 -> Add5/2
  Gain26/1 -> Add4/2
  Fcn23/1 -> Gain25/1
  Fcn26/1 -> Gain28/1
  Constant5/1 -> Add5/6
  Fcn20/1 -> Gain18/1
  Add4/1 -> dq2d/1
  Add3/1 -> dq1d/1
  Add5/1 -> dq3d/1
  Fcn22/1 -> Gain20/1
  Fcn27/1 -> Gain15/1
  Fcn30/1 -> Gain23/1
  Gain17/1 -> Add5/1
  Gain24/1 -> Add3/5
  Constant3/1 -> Add3/6
  Gain16/1 -> Add3/2
  Gain22/1 -> Add3/3
  Fcn19/1 -> Gain17/1
  Gain15/1 -> Add3/1
  Gain23/1 -> Add3/4
  Fcn29/1 -> Gain22/1
  Gain29/1 -> Add4/5
  Fcn17/1 -> Gain24/1
  Fcn24/1 -> Gain26/1
  Gain25/1 -> Add4/1
  Fcn25/1 -> Gain27/1
  Fcn28/1 -> Gain16/1
  Constant4/1 -> Add4/6
  Gain28/1 -> Add4/4
  Fcn16/1 -> Gain29/1
  Gain27/1 -> Add4/3
  Merge/1 -> Fcn33/1, Fcn37/1, Fcn36/1, Fcn35/1, Fcn34/1, Fcn31/1, Fcn41/1, Fcn40/1, Fcn39/1, Fcn38/1, Fcn32/1, Fcn45/1, Fcn44/1, Fcn43/1, Fcn42/1, Fcn18/1, Fcn22/1, Fcn21/1, Fcn20/1, Fcn19/1, Fcn16/1, Fcn26/1, Fcn25/1, Fcn24/1, Fcn23/1, Fcn17/1, Fcn30/1, Fcn29/1, Fcn28/1, Fcn27/1, Fcn11/1, Fcn15/1, Fcn14/1, Fcn13/1, Fcn12/1, Fcn1/1, Fcn5/1, Fcn4/1, Fcn3/1, Fcn2/1, Fcn10/1, Fcn9/1, Fcn8/1, Fcn7/1, Fcn6/1
  Gain32/1 -> Add8/1
  Gain39/1 -> Add6/5
  Constant6/1 -> Add6/6
  Fcn45/1 -> Gain38/1
  Add7/1 -> ddq2d/1
  Fcn42/1 -> Gain30/1
  Add8/1 -> ddq3d/1
  Fcn35/1 -> Gain33/1
  Gain41/1 -> Add7/2
  Fcn37/1 -> Gain35/1
  Gain36/1 -> Add8/5
  Gain35/1 -> Add8/4
  Fcn36/1 -> Gain34/1
  Gain34/1 -> Add8/3
  Fcn33/1 -> Gain36/1
  Gain42/1 -> Add7/3
  Fcn39/1 -> Gain41/1
  Gain33/1 -> Add8/2
  Gain43/1 -> Add7/4
  Add6/1 -> ddq1d/1
  Gain40/1 -> Add7/1
  Constant8/1 -> Add8/6
  Constant7/1 -> Add7/6
  Fcn41/1 -> Gain43/1
  Fcn43/1 -> Gain31/1
  Fcn38/1 -> Gain40/1
  Fcn40/1 -> Gain42/1
  Fcn31/1 -> Gain44/1
  Gain38/1 -> Add6/4
  Fcn44/1 -> Gain37/1
  Fcn34/1 -> Gain32/1
  Gain37/1 -> Add6/3
  Gain30/1 -> Add6/1
  Gain31/1 -> Add6/2
  Gain44/1 -> Add7/5
  Fcn32/1 -> Gain39/1
  Constant9/1 -> If Action Subsystem1/1(In1), If/2
  If/1 -> If Action Subsystem/Action
  If/2 -> If Action Subsystem1/Action
  If Action Subsystem1/1(Out1) -> Merge/2
  If Action Subsystem/1(Out1) -> Merge/1
  thetad/1 -> Terminator/1
  theta_init/1 -> Terminator1/1

== system backup_of_step3/Trajectory Planning Module/If Action Subsystem ==
  In1 : Inport
  Action Port : ActionPort  ActionPortLabel=if(u1 < t_action)
  Out1 : Outport
  wires:
  In1/1 -> Out1/1

== system backup_of_step3/Trajectory Planning Module/If Action Subsystem1 ==
  In1 : Inport
  Action Port : ActionPort  ActionPortLabel=else
  Out1 : Outport
  wires:
  In1/1 -> Out1/1

== matlab function Subsystem1/MATLAB Function ==
  data: F input double; thetaF input double; Tau1 output double; Mz input double; Rparams input double; q input double; Tau2 output double; Tau3 output double
function [Tau1,Tau2, Tau3] = fcn(F, thetaF, Mz, Rparams, q)

m = Rparams(1);
L = Rparams(2);
gama0 = Rparams(3);
gama1 = Rparams(4);
gama2 = Rparams(5);
gama3 = Rparams(6);


FxL = F*L*cos(thetaF);
FyL = F*L*sin(thetaF);
F_cartesian = [FxL; FyL; Mz];

Rparams4J = zeros(4);
Rparams4J(1) = gama1;
Rparams4J(2) = gama2;
Rparams4J(3) = gama3;
Rparams4J(4) = L;
J = PRBDM_3R_Jacobi(q,Rparams4J);

J_T = transpose(J);

Tau = J_T*F_cartesian;
Tau1 = Tau(1);
Tau2 = Tau(2);
Tau3 = Tau(3);

== matlab function Subsystem/MATLAB Function ==
  data: F input double; thetaF input double; Tau1 output double; Mz input double; Rparams input double; q input double; Tau2 output double; Tau3 output double
function [Tau1,Tau2, Tau3] = fcn(F, thetaF, Mz, Rparams, q)

m = Rparams(1);
L = Rparams(2);
gama0 = Rparams(3);
gama1 = Rparams(4);
gama2 = Rparams(5);
gama3 = Rparams(6);


FxL = F*L*cos(thetaF);
FyL = F*L*sin(thetaF);
F_cartesian = [FxL; FyL; Mz];

Rparams4J = zeros(4);
Rparams4J(1) = gama1;
Rparams4J(2) = gama2;
Rparams4J(3) = gama3;
Rparams4J(4) = L;
J = PRBDM_3R_Jacobi(q,Rparams4J);

J_T = transpose(J);

Tau = J_T*F_cartesian;
Tau1 = Tau(1);
Tau2 = Tau(2);
Tau3 = Tau(3);
